simulink model "logicRefChapter3"  (R2022b)
settings: Solver=ode45  StartTime=0.0  StopTime=10.0  RelTol=1e-3  EnableMultiTasking=on
PreLoadFcn:
  | % Input Data
  | etc_logic_data;
values from neighbouring files (symbols this model uses):
  Ts = 0.01    [allParamValues.mat]
settings Model: Creator=nicholas  LastModifiedBy=bensweet
settings SolverCC: MaxConsecutiveZCs=25  AlgebraicLoopSolver=TrustRegion
settings DataIOCC: LimitDataPoints=on  SaveFormat=Array  ReturnWorkspaceOutputs=off
settings OptimizationCC: DefaultParameterBehavior=Inlined  ExpressionDepthLimit=2147483647  InitFltsAndDblsToZero=on  LifeSpan=inf
settings DebuggingCC: UnconnectedInputMsg=warning  UnconnectedOutputMsg=warning  UnconnectedLineMsg=warning  PregeneratedLibrarySubsystemCodeDiagnostic=none  SFMachineParentedDataDiag=warning
settings HardwareCC: ProdBitPerPointer=32  ProdBitPerSizeT=32  ProdBitPerPtrDiffT=32  ProdLargestAtomicFloat=None  ProdIntDivRoundTo=Undefined  ProdEndianess=Unspecified  ProdWordSize=32  ProdHWDeviceType=32-bit Generic
settings ModelReferenceCC: EnableRefExpFcnMdlSchedulingChecks=on  PropagateSignalLabelsOutOfModel=off
settings SFSimCC: SimUseLocalCustomCode=off
settings RTWCC: RTWUseLocalCustomCode=off  DLArmComputeVersion=19.05
settings CodeAppCC: StateflowObjectComments=on
settings GRTTargetCC: TargetLangStandard=C89/C90 (ANSI)  CombineOutputUpdateFcns=off  GRTInterface=on
settings ConfigComp: CovMetricSettings=dw  CovSaveCumulativeToWorkspaceVar=on  CovSaveSingleToWorkspaceVar=on  CovExternalEMLEnable=off  CovSFcnEnable=off

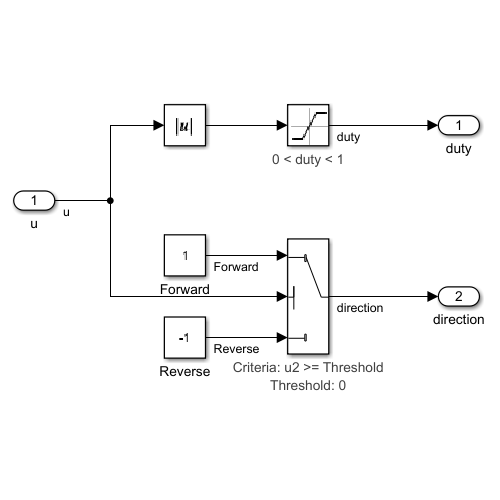
[thumbnail: Simulink's stored preview of the top-level diagram]
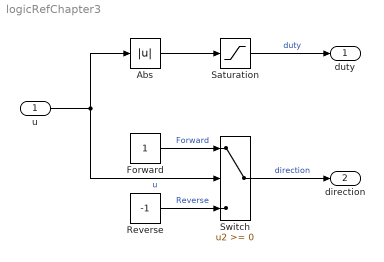
== system logicRefChapter3 ==
  u : Inport  SampleTime=Ts
  Abs : Abs  SaturateOnIntegerOverflow=off
  Forward : Constant  OutDataTypeStr=double
  Reverse : Constant  Value=-1  OutDataTypeStr=double
  Saturation : Saturate  UpperLimit=1  LowerLimit=0
      settings: AttributesFormatString=%<LowerLimit> < duty < %<UpperLimit>
  Switch : Switch  SaturateOnIntegerOverflow=off  InputSameDT=off
      settings: AttributesFormatString=Criteria: %<Criteria>\nThreshold: %<Threshold>
  duty : Outport  SampleTime=Ts  VectorParamsAs1DForOutWhenUnconnected=off
  direction : Outport  Port=2  SampleTime=Ts  VectorParamsAs1DForOutWhenUnconnected=off
  wires:
  Abs/1 -> Saturation/1
  Saturation/1 -> duty/1  "duty"
  Switch/1 -> direction/1  "direction"
  Reverse/1 -> Switch/3  "Reverse"
  Forward/1 -> Switch/1  "Forward"
  u/1 -> Switch/2, Abs/1  "u"
